simulink model "Function11"  (R2020b)
settings: Solver=VariableStepAuto  StartTime=0.0  StopTime=10.0  RelTol=1e-3
libraries: simulink x3
settings Model: Creator=viett  LastModifiedBy=ASUS
settings DataIOCC: ReturnWorkspaceOutputs=off
settings DebuggingCC: ArithmeticOperatorsInVariantConditions=warning
settings SFSimCC: SimUseLocalCustomCode=off  CustomCodeUndefinedFunction=UseInterfaceOnly
settings RTWCC: RTWUseLocalCustomCode=off
settings CodeAppCC: StateflowObjectComments=on

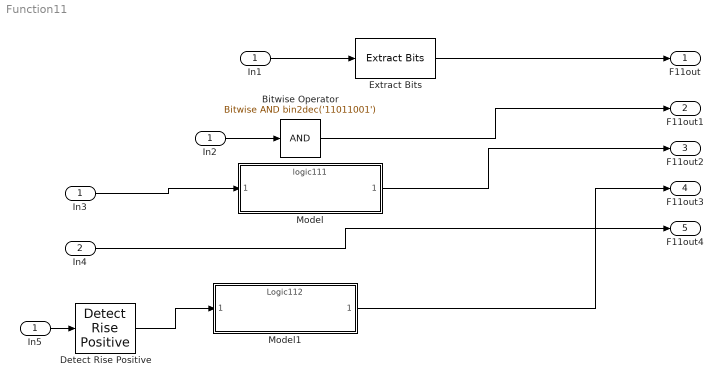
== system Function11 ==
  In1 : Inport
  In4 : Inport  Port=2
  Bitwise Operator : simulink/Logic and Bit Operations/Bitwise Operator  logicop=AND  UseBitMask=on  BitMask=bin2dec('11011001')  BitMaskRealWorld=Stored Integer
  Detect Rise Positive : simulink/Logic and Bit Operations/Detect Rise Positive  vinit=0  OutDataTypeStr=boolean
  Extract Bits : simulink/Logic and Bit Operations/Extract Bits  bitsToExtract=Upper half  numBits=8  bitIdxRange=[0 7]  outScalingMode=Preserve fixed-point scaling
  In2 : InportShadow
  In3 : InportShadow
  In5 : InportShadow
  Model : ModelReference  ModelNameDialog=logic111.slx  SimulationMode=Normal  ModelReferenceVersion=1.8
  Model1 : ModelReference  ModelNameDialog=Logic112  SimulationMode=Normal  ModelReferenceVersion=1.2
  F11out : Outport
  F11out1 : Outport  Port=2
  F11out2 : Outport  Port=3
  F11out3 : Outport  Port=4
  F11out4 : Outport  Port=5
  wires:
  Extract Bits/1 -> F11out/1
  Model/1 -> F11out2/1
  Bitwise Operator/1 -> F11out1/1
  Model1/1 -> F11out3/1
  Detect Rise Positive/1 -> Model1/1
  In1/1 -> Extract Bits/1
  In2/1 -> Bitwise Operator/1
  In3/1 -> Model/1
  In5/1 -> Detect Rise Positive/1
  In4/1 -> F11out4/1
